simulink model "VehiclePlant"  (R2020a)
settings: Solver=VariableStepAuto  StartTime=0.0  StopTime=10.0  RelTol=1e-3
libraries: mpclib x2
settings Model: Creator=francesco  LastModifiedBy=francesco

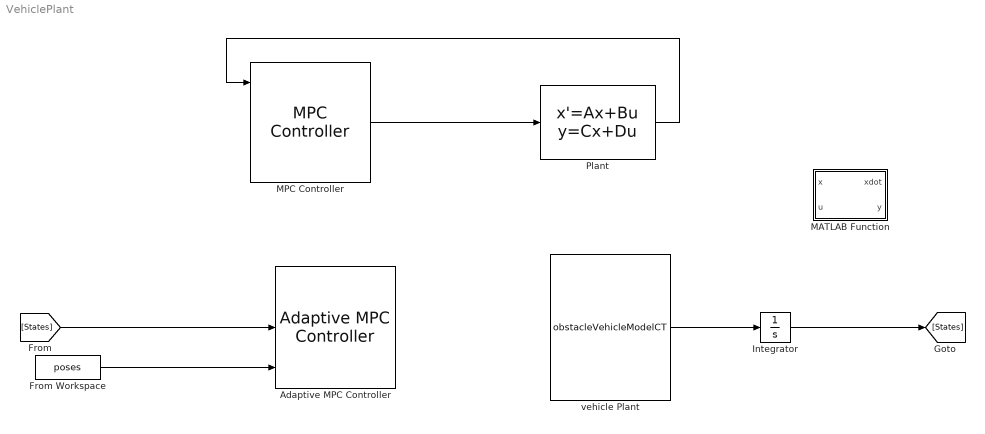
== system VehiclePlant ==
  Adaptive MPC Controller : mpclib/Adaptive MPC Controller  SCDEnableBlockLinearizationSpecification=on  enable_value=0  updateMPCinCallerWorkspace=on  md_inport=off  mv_inport=off  uref_inport=off  return_cost=off  return_mvseq=off  return_qpstatus=off  return_xseq=off  return_state=off  return_ovseq=off  state_inport=off  isltv_plant=off  umin_inport=off  umax_inport=off  ymin_inport=off  ymax_inport=off  cc_inport=off  ywt_inport=off  uwt_inport=off  duwt_inport=off  rhoeps_inport=off  pm_inport=off  MaximumP=10  HorizonChoice=FixedHorizon  BlockDataType=double  SampleTimeInherited=off  switch_inport=off
  From Workspace : FromWorkspace  VariableName=poses
  Integrator : Integrator
  MATLAB Function : MATLAB Function  TreatAsAtomicUnit=on
  MPC Controller : mpclib/MPC Controller  SCDEnableBlockLinearizationSpecification=on  is_multiple=0  enable_value=0  return_u0=off  updateMPCinCallerWorkspace=on  md_inport=on  mv_inport=off  uref_inport=off  return_cost=off  return_mvseq=off  return_qpstatus=off  return_xseq=off  return_state=off  return_ovseq=off  state_inport=off  umin_inport=off  umax_inport=off  ymin_inport=off  ymax_inport=off  cc_inport=off  ywt_inport=off  uwt_inport=off  duwt_inport=off  rhoeps_inport=off  pm_inport=off  MaximumP=10  HorizonChoice=FixedHorizon  n_ts=1  n_p=10  n_mv=1  n_md=1  n_ud=0  n_mo=1  n_uo=0  BlockDataType=double  SampleTimeInherited=off  switch_inport=off
  Plant : StateSpace  A=|  B=|  C=[1 0 0 0; 0 1 0 0; 0 0 1 0; 0 0 0 1]  D=0  InitialCondition=0  ContinuousStateAttributes='xPos', 'yPos', 'theta', 'v'
      A=|
      | [ 0, 0, -x(4)*sin(x(3)), cos(x(3));
      |       0, 0,  x(4)*cos(x(3)), sin(x(3));
      |       0, 0, 0,             tan(x(3))/carLength;
      |       0, 0, 0,             0]
      B=|
      | [0  , 0;
      |      0  , 0;
      |      0  , (x(4)*(tan(x(3))^2 + 1))/carLength;
      |      0.5, 0];
  vehicle Plant : Fcn  Expr=obstacleVehicleModelCT
  wires:
  MPC Controller/1 -> Plant/1
  Plant/1 -> MPC Controller/1
  vehicle Plant/1 -> Integrator/1
  From Workspace/1 -> Adaptive MPC Controller/3
  Integrator/1 -> [States]
  [States] -> Adaptive MPC Controller/2

== matlab function VehiclePlant/MATLAB Function ==
  data: x input; xdot output; u input; y output
function [xdot,y] = obstacleVehicleModelCT(x,u)
% The ego car has rectangular shaper with a length of 5 meters and width of
% 2 meters. The model has four states:
%
% * |xPos| - Global horizontal position of the car center
% * |yPos| - Global vertical position of the car center
% * |theta| - Heading angle of the car (0 when facing east, counterclockwise positive)
% * |V| - Speed of the car (positve)
%
% There are two manipulated variables:
%
% * |throttle| - Throttle (positive when accelerating, negative when braking)
% * |delta| - Steering angle change (counterclockwise positive)
%

%#codegen
carLength = egoVehicle.Length;
theta = x(3);
V = x(4);
delta = u(2);
A = [ 0, 0, -V*sin(theta), cos(theta);
      0, 0,  V*cos(theta), sin(theta);
      0, 0, 0,             tan(delta)/carLength;
      0, 0, 0,             0];
B = [0  , 0;
     0  , 0;
     0  , (V*(tan(delta)^2 + 1))/carLength;
     0.5, 0];
C = eye(4);
D = zeros(4,2);
xdot = A*x + B*u;
y = C*x + D*u;
